simulink model "F16ASYM_Controlled"  (R2015a)
settings: Solver=ode3  SolverMode=SingleTasking  StartTime=0.0  StopTime=inf  FixedStep=T_sim  RelTol=1e-3
InitFcn:
  | load('NN_c_weights_Last_stable.mat')
StopFcn:
  | Final_results
values from neighbouring files (symbols this model uses):
  a1 = fitresult.p1    [Stall_protection.m]
  alpha_map_eval = ones(size(M_eval))*NaN    [Auto_trim_aid.m]    (also in Autotrim_maps.mat = [nan nan 0.277598136245 0.119432432992 0.0579479097061 0.027)
  beta_map_eval = ones(size(M_eval))*NaN    [Auto_trim_aid.m]    (also in Autotrim_maps.mat = [nan nan -0.00151549403324 0.00117807579006 -0.0052086799721)
  C_L_0 = fitresult.p2    [Stall_protection.m]
  G_eval = NaN*ones(size(M_sq,2),size(H_sq,2))    [Stall_protection.m]
  H_sq = unique(sort(H_sq))    [Stall_protection.m]
  H_sq_autotrim = min( F_envelope.H_1g):2000:max(F_envelope.H_1g)    [Auto_trim_aid.m]    (also in Autotrim_maps.mat = [0 2000 4000 6000 8000 10000 12000 14000 16000 18000])
  K_b_q_extrap_ACC = K_b_q_extrap    [RUN_ME.m]
  K_b_q_extrap_AoA = K_b_q_extrap    [RUN_ME.m]
  M_sq = unique(sort(M_sq))    [Stall_protection.m]
  M_sq_autotrim = 0:0.1:max(F_envelope.M_1g)    [Auto_trim_aid.m]    (also in Autotrim_maps.mat = [0 0.1 0.2 0.3 0.4 0.5 0.6 0.7 0.8 0.9 1 1.1 ... (21 element)
  T_sim = 0.02    [RUN_ME.m]
  tau_q_extrap_ACC = tau_q_extrap    [RUN_ME.m]
  tau_q_extrap_AoA = tau_q_extrap    [RUN_ME.m]
  velocity = M_eval(I,J)*a    [Auto_trim_aid.m]
undefined symbols (not defined in the file or in its folder): ACCEL, B, Earth, fi_flag_Simulink, GYRO, H_sq_sche, k_B, K_b_ACC_extrap, K_b_AoA_extrap, latitude, longitude, m, m_B, M_sq_sche, Model_used_flag, rad, s, sigbuilder_block, Stall_curve, tau_ACC_extrap, tau_AoA_extrap, Theta_1_roll_last, Theta_2_roll_last, Theta_3_roll_last, trim_control, trim_state, trim_throttle, V_Comp_A_w_z_last, V_Comp_last, V_Comp_last_ONE, V_long_lastA_w_z, V_long_lastAoA, V_roll_last, V_roll_lastMOD, V_yaw_last, W_Comp_A_w_z_last, W_Comp_last, W_long_lastA_w_z, W_long_lastAoA, W_roll_last, W_roll_lastMOD, W_yaw_last, WGS84
libraries: Adaptive_FaultTolerantControl x57, dspsigops x37, F16_Actuator_Library x14, commnoisgen2 x13, simulink x11, simulink_extras x10, dsparch4 x6, aerolibatmos2 x6, aerolibtransform2 x6, aerolibfltsims x3, dspvision x3, dspsnks4 x3
(part 3 of 14)

== system F16ASYM_Controlled/NDI/NDI: NO RECONFIG ==
  note: These two block MUST be evaluated at the same dynamics X
      | and control deflections delta*
      |
      |
      | delta* are a given set of control deflection: can be either the initial trim set
      | or the previous deflections
  Est reconf : Inport
  Angular_acc_des (rad/s^2) : Inport  Port=2
  All_meas : Inport  Port=3
  Control_defl for eval : Inport  Port=4
  Bus Selector : BusSelector  OutputSignals=signal1.omega_b meas (rad/s),signal2.q (Pa),signal1.Alt meas (m),signal1.V_TAS (m/s),signal1.AoA meas (rad),signal1.SS meas (rad),signal1.Throttle_meas
  Demux : Demux  Outputs=3
  Dim_less : Subsystem
  Inversion : Sum  Inputs=|+-
  Memory : Memory  X0=[0,0,0]
  Mom Coefficients gradient with control deflections at the given dynamics X: It performs perturbations theory arroun the given control deflections : MATLABFcn  MATLABFcn=Moms_Coeff_Grad_estimator  OutputDimensions=21  OutputSignalType=real
  Mux : Mux  Inputs=3
  Mux1 : Mux  Inputs=7
  Pre-Inverter : MATLAB Function  TreatAsAtomicUnit=on
  Reshape : Reshape  OutputDimensionality=Customize  OutputDimensions=[k_B,m_B]
  Terminator : Terminator
  Trim controls Asym In LEFs: Additionaly from dLEF : Constant  Commented=on  Value=[trim_control(1),trim_control(1),trim_control(2),-trim_control(2),trim_control(3),0,0]
  "f(x)  Mom Coefficients due to the dynamics: Coefficients model with control inputs " : MATLABFcn  MATLABFcn=Moms_Coeff_estimator  OutputDimensions=3  OutputSignalType=real
  Virtual Control Commands : Outport
  B online : Outport  Port=2
  Control_defl evald : Outport  Port=3
  Mom coef comm : Outport  Port=4
  wires:
  Est reconf/1 -> Terminator/1
  Reshape/1 -> B online/1
  Mom Coefficients gradient with control deflections at the given dynamics X: It performs perturbations theory arroun the given control deflections/1 -> Reshape/1
  Mux/1 -> Memory/1, Inversion/1
  Bus Selector/7 -> Mux1/6  "<Throttle_meas>"
  Mux1/1 -> Mom Coefficients gradient with control deflections at the given dynamics X: It performs perturbations theory arroun the given control deflections/1, "f(x)  Mom Coefficients due to the dynamics: Coefficients model with control inputs "/1
  Control_defl for eval/1 -> Mux1/7, Control_defl evald/1
  Bus Selector/6 -> Mux1/4  "<SS meas (rad)>"
  Bus Selector/5 -> Mux1/3  "<AoA meas (rad)>"
  Bus Selector/4 -> Mux1/2  "<V_TAS (m/s)>"
  Bus Selector/3 -> Mux1/1  "<Alt meas (m)>"
  "f(x)  Mom Coefficients due to the dynamics: Coefficients model with control inputs "/1 -> Inversion/2  "f(x) or C_x"
  Dim_less/3(C_N des) -> Mux/3
  Dim_less/2(C_M des) -> Mux/2
  Dim_less/1(C_L des) -> Mux/1
  Pre-Inverter/3(N_comm) -> Dim_less/3(N_comm)
  Pre-Inverter/2(M_comm) -> Dim_less/2(M_comm)
  Pre-Inverter/1(L_comm) -> Dim_less/1(L_comm)
  Bus Selector/2 -> Dim_less/4(q)  "<q (Pa)>"
  All_meas/1 -> Bus Selector/1
  Demux/1 -> Pre-Inverter/1(p_dot_comm)
  Demux/3 -> Pre-Inverter/3(r_dot_comm)
  Demux/2 -> Pre-Inverter/2(q_dot_comm)
  Angular_acc_des (rad/s^2)/1 -> Demux/1
  Bus Selector/1 -> Mux1/5, Pre-Inverter/4(omega_b)  "<omega_b meas (rad/s)>"
  Inversion/1 -> Virtual Control Commands/1
  Memory/1 -> Mom coef comm/1

== system F16ASYM_Controlled/NDI/NDI: RECONFIG ==
  note: These two block MUST be evaluated at the same dynamics X
      | and control deflections delta*
      |
      |
      | delta* are a given set of control deflection: can be either the initial trim set
      | or the previous deflections
  note: INPUTS
      | States:
      |
      | 1. Altitude
      | 2. TAS velocity
      | 3. alpha in rad
      | 4. beta in rads
      | 5. P
      | 6. Q
      | 7. R
      | 8. Throttle
      | 9. Elevator_L in deg
      | 10. Elevator_R in deg
      | 11. Aileron_L
      | 12. Aileron_R
      | 13. Rudder
      | 14. LEF_L
      | 15. LEF_R
      |
      | RECONFIGURATION PARAMETERS
      |
      | 16. mass  Estimated mass
      | 17. S_current_L
      | 18. S_current_R
      | 19. S_fin_current
      | 20. x_cg
      | 21. Jy
      | 22. Jxz
      | 23. Jz
      | 24. Jx
      | 25. EFF_el_L
      | 26. EFF_el_R
      | 27. EFF_ail_L
      | 28 EFF_ail_R
      | 29. EFF_rud
      | 30. EFF_lef_L
      | 31. EFF_lef_R
      | 32. Delta_C_Lift_X
      | 33. Delta_C_Drag_X
      | 34. Delta_C_m_X
  Est reconf : Inport
  Angular_acc_des (rad/s^2) : Inport  Port=2
  All_meas : Inport  Port=3
  Control_defl for eval : Inport  Port=4
  Bus Selector : BusSelector  OutputSignals=signal1.omega_b meas (rad/s),signal2.q (Pa),signal1.Alt meas (m),signal1.V_TAS (m/s),signal1.AoA meas (rad),signal1.SS meas (rad),signal1.Throttle_meas
  Bus Selector1 : BusSelector  OutputSignals=Reconfig signal
  Controls : Scope
      settings: SaveName=ScopeData19
  Demux : Demux  Outputs=3
  Dim_less : Subsystem
  Inversion : Sum  Inputs=|+-
  Memory : Memory  X0=[0,0,0]
  Mom Coefficients gradient with control deflections at the given dynamics X: It performs perturbations theory arroun the given control deflections : MATLABFcn  MATLABFcn=Moms_Coeff_Grad_Reconf_estimator  OutputDimensions=21  OutputSignalType=real
  Mux : Mux  Inputs=3
  Mux1 : Mux  Inputs=7
  Mux2 : Mux  Inputs=[15 19]
  Plant : Scope
      settings: SaveName=ScopeData11
  Pre-Inverter : MATLAB Function  TreatAsAtomicUnit=on
  Reshape : Reshape  OutputDimensionality=Customize  OutputDimensions=[k_B,m_B]
  Signal Specification : SignalSpecification  Dimensions=19
  Trim controls Asym In LEFs: Additionaly from dLEF : Constant  Commented=on  Value=[trim_control(1),trim_control(1),trim_control(2),-trim_control(2),trim_control(3),0,0]
  f(x)  Mom Coefficients due to the dynamics: Coefficients model with control inputs : MATLABFcn  MATLABFcn=Moms_Coeff_Reconf_estimator  OutputDimensions=3  OutputSignalType=real
  Virtual Control Commands : Outport
  B online : Outport  Port=2
  Control_defl evald : Outport  Port=3
  Mom coef comm : Outport  Port=4
  wires:
  Inversion/1 -> Controls/1, Virtual Control Commands/1
  Bus Selector/1 -> Pre-Inverter/4(omega_b), Mux1/5  "<omega_b meas (rad/s)>"
  Angular_acc_des (rad/s^2)/1 -> Demux/1
  Demux/2 -> Pre-Inverter/2(q_dot_comm)
  Demux/3 -> Pre-Inverter/3(r_dot_comm)
  Demux/1 -> Pre-Inverter/1(p_dot_comm)
  All_meas/1 -> Bus Selector/1
  Bus Selector/2 -> Dim_less/4(q)  "<q (Pa)>"
  Pre-Inverter/1(L_comm) -> Dim_less/1(L_comm)
  Pre-Inverter/2(M_comm) -> Dim_less/2(M_comm)
  Pre-Inverter/3(N_comm) -> Dim_less/3(N_comm)
  Dim_less/1(C_L des) -> Mux/1
  Dim_less/2(C_M des) -> Mux/2
  Dim_less/3(C_N des) -> Mux/3
  f(x)  Mom Coefficients due to the dynamics: Coefficients model with control inputs/1 -> Plant/1, Inversion/2  "f(x) or C_x"
  Bus Selector/3 -> Mux1/1  "<Alt meas (m)>"
  Bus Selector/4 -> Mux1/2  "<V_TAS (m/s)>"
  Bus Selector/5 -> Mux1/3  "<AoA meas (rad)>"
  Bus Selector/6 -> Mux1/4  "<SS meas (rad)>"
  Control_defl for eval/1 -> Mux1/7, Control_defl evald/1
  Bus Selector/7 -> Mux1/6  "<Throttle_meas>"
  Mux/1 -> Inversion/1, Memory/1
  Mom Coefficients gradient with control deflections at the given dynamics X: It performs perturbations theory arroun the given control deflections/1 -> Reshape/1
  Reshape/1 -> B online/1
  Est reconf/1 -> Bus Selector1/1
  Bus Selector1/1 -> Signal Specification/1  "<Reconfig signal>"
  Mux1/1 -> Mux2/1
  Mux2/1 -> Mom Coefficients gradient with control deflections at the given dynamics X: It performs perturbations theory arroun the given control deflections/1, f(x)  Mom Coefficients due to the dynamics: Coefficients model with control inputs/1
  Signal Specification/1 -> Mux2/2
  Memory/1 -> Mom coef comm/1

== system F16ASYM_Controlled/Primary Controller/P con  + Crossed NN + AWU+Lim + hand-over+Scheduling ==
  note: Indicator correspond to 0
  note: Indicator correspond to 1
  A_w_z des : Inport
  AoA des (rad) : Inport  Port=2
  p des (rad/s) : Inport  Port=3
  beta des (rad) : Inport  Port=4
  Anti-windup A_w_z : Inport  Port=5
  Anti-windup AoA : Inport  Port=6
  Anti-windup beta : Inport  Port=7
  All measures : Inport  Port=8
  Anti-windup signals : Inport  Port=9
  A_w_z des1 : InportShadow
  Anti-windup A_w_z1 : InportShadow  Port=5
  Anti-windup AoA1 : InportShadow  Port=6
  Anti-windup beta1 : InportShadow  Port=7
  Anti-windup signals1 : InportShadow  Port=9
  AoA des (rad)1 : InportShadow  Port=2
  Bus Selector : BusSelector  OutputSignals=signal2.a,signal1.V_TAS (m/s)
  Gain2 : Gain  Gain=2
  Logical Operator : Logic  Operator=NOT  IconShape=distinctive  AllPortsSameDT=off  OutDataTypeStr=boolean
  Min TAS : Product  Inputs=**
  "P controller + adaptive Crossed NN + AWU+Lim    in ACC " : Subsystem  VariantControl=Adaptive Controller Crossed+AWU+Lim
  P controller + adaptive Crossed NN + AWU+Lim   in AoA : Subsystem  VariantControl=Adaptive Controller Crossed+AWU+Lim
  Relational Operator5 : RelationalOperator  OutDataTypeStr=boolean
  "Transitions Smoother " : Subsystem
  beta des (rad)1 : InportShadow  Port=4
  p des (rad/s)1 : InportShadow  Port=3
  Angular acc des : Outport
  Control_in : Outport  Port=2
  wires:
  Logical Operator/1 -> "P controller + adaptive Crossed NN + AWU+Lim    in ACC "/10(Active)
  "Transitions Smoother "/1(Ang accels comm) -> Angular acc des/1
  Relational Operator5/1 -> P controller + adaptive Crossed NN + AWU+Lim   in AoA/10(Active), Control_in/1, "Transitions Smoother "/2(Indicator), Logical Operator/1
  P controller + adaptive Crossed NN + AWU+Lim   in AoA/1(Angular acc des) -> "Transitions Smoother "/1(From AoA)
  "P controller + adaptive Crossed NN + AWU+Lim    in ACC "/1(Angular acc des) -> "Transitions Smoother "/3(From  ACC)
  Bus Selector/2 -> Relational Operator5/2  "<V_TAS (m/s)>"
  Gain2/1 -> Relational Operator5/1
  Min TAS/1 -> Gain2/1
  Bus Selector/1 -> Min TAS/2  "<a>"
  [Min_Mach] -> Min TAS/1  "Min M"
  Anti-windup signals1/1 -> "P controller + adaptive Crossed NN + AWU+Lim    in ACC "/9(Anti-windup signals)
  All measures/1 -> P controller + adaptive Crossed NN + AWU+Lim   in AoA/8(All measures), Bus Selector/1, "P controller + adaptive Crossed NN + AWU+Lim    in ACC "/8(All measures)
  Anti-windup beta1/1 -> "P controller + adaptive Crossed NN + AWU+Lim    in ACC "/7(Anti-windup beta)
  Anti-windup AoA1/1 -> "P controller + adaptive Crossed NN + AWU+Lim    in ACC "/6(Anti-windup AoA)
  Anti-windup A_w_z1/1 -> "P controller + adaptive Crossed NN + AWU+Lim    in ACC "/5(Anti-windup A_w_z)
  beta des (rad)1/1 -> "P controller + adaptive Crossed NN + AWU+Lim    in ACC "/4(beta des (rad))
  p des (rad/s)1/1 -> "P controller + adaptive Crossed NN + AWU+Lim    in ACC "/3(p des (rad/s))
  AoA des (rad)1/1 -> "P controller + adaptive Crossed NN + AWU+Lim    in ACC "/2(AoA des (rad))
  A_w_z des1/1 -> "P controller + adaptive Crossed NN + AWU+Lim    in ACC "/1(A_w_z des)
  p des (rad/s)/1 -> P controller + adaptive Crossed NN + AWU+Lim   in AoA/3(p des (rad/s))
  beta des (rad)/1 -> P controller + adaptive Crossed NN + AWU+Lim   in AoA/4(beta des (rad))
  AoA des (rad)/1 -> P controller + adaptive Crossed NN + AWU+Lim   in AoA/2(AoA des (rad))
  Anti-windup AoA/1 -> P controller + adaptive Crossed NN + AWU+Lim   in AoA/6(Anti-windup AoA)
  Anti-windup A_w_z/1 -> P controller + adaptive Crossed NN + AWU+Lim   in AoA/5(Anti-windup A_w_z)
  A_w_z des/1 -> P controller + adaptive Crossed NN + AWU+Lim   in AoA/1(A_w_z des)
  Anti-windup beta/1 -> P controller + adaptive Crossed NN + AWU+Lim   in AoA/7(Anti-windup beta)
  Anti-windup signals/1 -> P controller + adaptive Crossed NN + AWU+Lim   in AoA/9(Anti-windup signals)

== system F16ASYM_Controlled/Primary Controller/P con + Crossed NN + AWU+Lim + hand-over ==
  note: Indicator correspond to 1
  note: Indicator correspond to 0
  A_w_z des : Inport
  AoA des (rad) : Inport  Port=2
  p des (rad/s) : Inport  Port=3
  beta des (rad) : Inport  Port=4
  Anti-windup A_w_z : Inport  Port=5
  Anti-windup AoA : Inport  Port=6
  Anti-windup beta : Inport  Port=7
  All measures : Inport  Port=8
  Anti-windup signals : Inport  Port=9
  A_w_z des1 : InportShadow
  Anti-windup A_w_z1 : InportShadow  Port=5
  Anti-windup AoA1 : InportShadow  Port=6
  Anti-windup beta1 : InportShadow  Port=7
  Anti-windup signals1 : InportShadow  Port=9
  AoA des (rad)1 : InportShadow  Port=2
  Bus Selector : BusSelector  OutputSignals=signal2.a,signal1.V_TAS (m/s)
  Gain2 : Gain  Gain=2
  Logical Operator : Logic  Operator=NOT  IconShape=distinctive  AllPortsSameDT=off  OutDataTypeStr=boolean
  Min TAS : Product  Inputs=**
  "P controller + adaptive Crossed NN + AWU+Lim    in ACC " : Subsystem  VariantControl=Adaptive Controller Crossed+AWU+Lim
  P controller + adaptive Crossed NN + AWU+Lim   in AoA : Subsystem  VariantControl=Adaptive Controller Crossed+AWU+Lim
  Relational Operator5 : RelationalOperator  OutDataTypeStr=boolean
  Scope : Scope
      settings: YMin=-2.75  YMax=0.25  SaveName=ScopeData32
  Scope1 : Scope  Commented=on
      settings: YMin=-2.75  YMax=0.25  SaveName=ScopeData33
  Switch : Switch  Commented=on  Threshold=0.5  InputSameDT=on
  Transition smoother : MATLAB Function  Commented=on  TreatAsAtomicUnit=on
  "Transitions Smoother " : Subsystem
  Transitions Smotother 1 : Subsystem  Commented=on
  Unit Delay : UnitDelay  Commented=on  SampleTime=-1
  beta des (rad)1 : InportShadow  Port=4
  p des (rad/s)1 : InportShadow  Port=3
  Angular acc des : Outport
  Control_in : Outport  Port=2
  wires:
  Anti-windup signals/1 -> P controller + adaptive Crossed NN + AWU+Lim   in AoA/9(Anti-windup signals)
  Anti-windup beta/1 -> P controller + adaptive Crossed NN + AWU+Lim   in AoA/7(Anti-windup beta)
  A_w_z des/1 -> P controller + adaptive Crossed NN + AWU+Lim   in AoA/1(A_w_z des)
  Anti-windup A_w_z/1 -> P controller + adaptive Crossed NN + AWU+Lim   in AoA/5(Anti-windup A_w_z)
  Anti-windup AoA/1 -> P controller + adaptive Crossed NN + AWU+Lim   in AoA/6(Anti-windup AoA)
  AoA des (rad)/1 -> P controller + adaptive Crossed NN + AWU+Lim   in AoA/2(AoA des (rad))
  beta des (rad)/1 -> P controller + adaptive Crossed NN + AWU+Lim   in AoA/4(beta des (rad))
  p des (rad/s)/1 -> P controller + adaptive Crossed NN + AWU+Lim   in AoA/3(p des (rad/s))
  A_w_z des1/1 -> "P controller + adaptive Crossed NN + AWU+Lim    in ACC "/1(A_w_z des)
  AoA des (rad)1/1 -> "P controller + adaptive Crossed NN + AWU+Lim    in ACC "/2(AoA des (rad))
  p des (rad/s)1/1 -> "P controller + adaptive Crossed NN + AWU+Lim    in ACC "/3(p des (rad/s))
  beta des (rad)1/1 -> "P controller + adaptive Crossed NN + AWU+Lim    in ACC "/4(beta des (rad))
  Anti-windup A_w_z1/1 -> "P controller + adaptive Crossed NN + AWU+Lim    in ACC "/5(Anti-windup A_w_z)
  Anti-windup AoA1/1 -> "P controller + adaptive Crossed NN + AWU+Lim    in ACC "/6(Anti-windup AoA)
  Anti-windup beta1/1 -> "P controller + adaptive Crossed NN + AWU+Lim    in ACC "/7(Anti-windup beta)
  All measures/1 -> "P controller + adaptive Crossed NN + AWU+Lim    in ACC "/8(All measures), Bus Selector/1, P controller + adaptive Crossed NN + AWU+Lim   in AoA/8(All measures)
  Anti-windup signals1/1 -> "P controller + adaptive Crossed NN + AWU+Lim    in ACC "/9(Anti-windup signals)
  [Min_Mach] -> Min TAS/1  "Min M"
  Bus Selector/1 -> Min TAS/2  "<a>"
  Min TAS/1 -> Gain2/1
  Gain2/1 -> Relational Operator5/1
  Bus Selector/2 -> Relational Operator5/2  "<V_TAS (m/s)>"
  "P controller + adaptive Crossed NN + AWU+Lim    in ACC "/1(Angular acc des) -> "Transitions Smoother "/3(From  ACC)
  P controller + adaptive Crossed NN + AWU+Lim   in AoA/1(Angular acc des) -> "Transitions Smoother "/1(From AoA)
  Relational Operator5/1 -> Logical Operator/1, Control_in/1, "Transitions Smoother "/2(Indicator), P controller + adaptive Crossed NN + AWU+Lim   in AoA/10(Active)
  Transition smoother/2(indicator_out) -> Unit Delay/1
  Unit Delay/1 -> Transition smoother/4(indicator_prev)
  "Transitions Smoother "/1(Ang accels comm) -> Angular acc des/1, Scope/1
  Switch/1 -> Scope1/1
  Logical Operator/1 -> "P controller + adaptive Crossed NN + AWU+Lim    in ACC "/10(Active)

== system F16ASYM_Controlled/Primary Controller/P con + adaptive Crossed NN + AWU+Lim + Scheduling ==
  A_w_z des : Inport
  AoA des (rad) : Inport  Port=2
  p des (rad/s) : Inport  Port=3
  beta des (rad) : Inport  Port=4
  Anti-windup A_w_z : Inport  Port=5
  Anti-windup AoA : Inport  Port=6
  Anti-windup beta : Inport  Port=7
  All measures : Inport  Port=8
  Anti-windup signals : Inport  Port=9
  Body Rates Controller : Subsystem  Variant=on  OverrideUsingVariant=Body rates controller of AoA
  Bus Creator : BusCreator  Inputs=3
  Bus Creator1 : BusCreator  Inputs=3
  Bus Creator2 : BusCreator
  Bus Creator3 : BusCreator  Inputs=2
  Bus Selector3 : BusSelector  OutputSignals=signal1.SS meas (rad)
  Complete crossed On-line (adaptive) multi-layer NN : Subsystem  Variant=on  OverrideUsingVariant=NN on AoA
      mask Display:
      | image(imread('ANN.png'))
      | 
      | port_label('input', 1, 'v prev')
      | port_label('input', 2, 'All meas')
      | port_label('input', 3, 'NN vars')
      | port_label('input', 4, 'Anti-windup')
      | 
      | port_label('output', 1, 'v_ad^')
  Constant : Constant  Value=NaN
  Display{,1..3,5..6} (6 alike) : Display
  "Display4 " : Display
  Lat_dir Dyn Inversion: beta_dot->r_c : Subsystem
  Long Dyn Inversion: alpha_dot ->q : Subsystem
  Longitudinal Controller: AoA or A_w_z : Subsystem  Variant=on  OverrideUsingVariant=Controller of AoA
  Memory : Memory  X0=[0,0,0]
  Physical limitation : Subsystem
  Ref Model and P Controller : Adaptive_FaultTolerantControl/Ref Model and P Controller  tau=0.45  y_i=trim_state(9)  K_f=1  K_b=5
  Scope1 : Scope
      settings: TimeRange=18  YMax=25  SaveName=ScopeData27
  Scope2 : Scope
      settings: TimeRange=18  YMax=25  SaveName=ScopeData7
  Scope3 : Scope
      settings: TimeRange=18  YMin=-20  YMax=1  SaveName=ScopeData21
  "Sigmoid " : Subsystem  mask{a=0.15}
      mask prompts: a "Sigmoid a param"
      mask TypeOptions a: a/Value
      mask Display:
      | x=-25:0.1:25;
      | 
      | y=(2.0 ./ (1.0 + exp(-a.*x))-1) ;
      | y2=zeros(size(x));
      | 
      | plot(x,y,x,y2);
      | 
      | text(-12,0.5, ['a= ',num2str(a)])
  Sum : Sum  Inputs=-+|
  Sum1 : Sum  Inputs=+-|
  Terminator1 : Terminator
  To Workspace : ToWorkspace  VariableName=Comm_ang_accel  SaveFormat=Timeseries  SampleTime=-1
  To Workspace1 : ToWorkspace  VariableName=NN_action  SaveFormat=Timeseries  SampleTime=-1
  Angular acc des : Outport
  Control_in : Outport  Port=2
  wires:
  Constant/1 -> Control_in/1
  Physical limitation/1(v limted) -> Angular acc des/1
  Anti-windup signals/1 -> Complete crossed On-line (adaptive) multi-layer NN/4(AWU)
  Ref Model and P Controller/1 -> Lat_dir Dyn Inversion: beta_dot->r_c/1(beta_dot_c), Display5/1
  Complete crossed On-line (adaptive) multi-layer NN/1(v_ad^) -> To Workspace1/1, Sum/1, Display2/1, Scope1/1  "v_ad^"
  "Sigmoid "/1(Out) -> Memory/1
  Anti-windup beta/1 -> Terminator1/1
  Bus Creator3/1 -> Bus Creator/3  "beta_r_chanel"
  Bus Creator2/1 -> Bus Creator3/2  "beta_chanel vars"
  Body Rates Controller/3(r_chanel vars) -> Bus Creator3/1  "r_chanel vars"
  Ref Model and P Controller/5 -> Bus Creator2/4  "K_b_beta"
  Ref Model and P Controller/4 -> Sum1/2
  Sum1/1 -> Bus Creator2/3  "beta_err"
  Ref Model and P Controller/3 -> Bus Creator2/2, Sum1/1  "beta_sf"
  Ref Model and P Controller/2 -> Bus Creator2/1  "beta_sf_dot"
  Bus Creator1/1 -> Bus Creator/1  "Long chanel"
  Longitudinal Controller: AoA or A_w_z/2(alpha_chanel vars) -> Bus Creator1/2  "alpha_chanel vars"
  Longitudinal Controller: AoA or A_w_z/1(A_chanel vars) -> Bus Creator1/1  "A_chanel vars"
  Body Rates Controller/1(q_chanel vars) -> Bus Creator1/3  "q_chanel_vars"
  Body Rates Controller/2(p_chanel vars) -> Bus Creator/2  "p_chanel_vars"
  Memory/1 -> Complete crossed On-line (adaptive) multi-layer NN/1(v_ad^ prev)
  Bus Creator/1 -> Complete crossed On-line (adaptive) multi-layer NN/3(NN variables)
  Body Rates Controller/4(Angular acc des (rad/s^2)) -> Scope2/1, Sum/2, Display3/1  "v_p+v_dot_ff"
  All measures/1 -> Longitudinal Controller: AoA or A_w_z/5(All meas), Long Dyn Inversion: alpha_dot ->q/2(All_meas), Bus Selector3/1, Lat_dir Dyn Inversion: beta_dot->r_c/2(All_meas), Body Rates Controller/4(All_meas), Physical limitation/2(all meas), Complete crossed On-line (adaptive) multi-layer NN/2(All_meas)
  Sum/1 -> To Workspace/1, Scope3/1, Physical limitation/1(v comm), "Sigmoid "/1(In), "Display4 "/1  "v"
  A_w_z des/1 -> Longitudinal Controller: AoA or A_w_z/1(A_w_z des)
  Anti-windup A_w_z/1 -> Longitudinal Controller: AoA or A_w_z/3(Anti-windup A_w_z)
  Anti-windup AoA/1 -> Longitudinal Controller: AoA or A_w_z/4(Anti-windup AoA)
  AoA des (rad)/1 -> Longitudinal Controller: AoA or A_w_z/2(AoA des (rad))
  Longitudinal Controller: AoA or A_w_z/3(alpha_dot_c) -> Display/1, Long Dyn Inversion: alpha_dot ->q/1(alpha_dot_c)
  beta des (rad)/1 -> Ref Model and P Controller/1
  Long Dyn Inversion: alpha_dot ->q/1(q_c) -> Display1/1, Body Rates Controller/2(q_ref)
  p des (rad/s)/1 -> Body Rates Controller/1(p_ref)
  Bus Selector3/1 -> Ref Model and P Controller/2  "<SS meas (rad)>"
  Lat_dir Dyn Inversion: beta_dot->r_c/1(r_c) -> Body Rates Controller/3(r_ref), Display6/1

== system F16ASYM_Controlled/Primary Controller/P cont + adaptive Crossed NN + AWU+Lim  ==
  A_w_z des : Inport
  AoA des (rad) : Inport  Port=2
  p des (rad/s) : Inport  Port=3
  beta des (rad) : Inport  Port=4
  Anti-windup A_w_z : Inport  Port=5
  Anti-windup AoA : Inport  Port=6
  Anti-windup beta : Inport  Port=7
  All measures : Inport  Port=8
  Anti-windup signals : Inport  Port=9
  Body Rates Controller : Subsystem
  Bus Creator : BusCreator  Inputs=3
  Bus Creator1 : BusCreator  Inputs=3
  Bus Creator2 : BusCreator
  Bus Creator3 : BusCreator  Inputs=2
  Bus Selector3 : BusSelector  OutputSignals=signal1.SS meas (rad)
  Complete crossed On-line (adaptive) multi-layer NN : Subsystem  Variant=on  OverrideUsingVariant=NN on AoA
      mask Display:
      | image(imread('ANN.png'))
      | 
      | port_label('input', 1, 'v prev')
      | port_label('input', 2, 'All meas')
      | port_label('input', 3, 'NN vars')
      | port_label('input', 4, 'Anti-windup')
      | 
      | port_label('output', 1, 'v_ad^')
  Constant : Constant  Value=NaN
  Display{,1..3,5..6} (6 alike) : Display
  "Display4 " : Display
  Lat_dir Dyn Inversion: beta_dot->r_c : Subsystem
  Long Dyn Inversion: alpha_dot ->q : Subsystem
  Longitudinal Controller: AoA or A_w_z : Subsystem  Variant=on  OverrideUsingVariant=Controller of AoA
  Memory : Memory  X0=[0,0,0]
  Physical limitation : Subsystem
  Ref Model and P Controller : Adaptive_FaultTolerantControl/Ref Model and P Controller  tau=0.8  y_i=trim_state(9)  K_f=1  K_b=5
  Scope1 : Scope
      settings: TimeRange=35  YMin=-0.0025  YMax=0.0275  SaveName=ScopeData27
  "Sigmoid " : Subsystem  mask{a=0.15}
      mask prompts: a "Sigmoid a param"
      mask TypeOptions a: a/Value
      mask Display:
      | x=-25:0.1:25;
      | 
      | y=(2.0 ./ (1.0 + exp(-a.*x))-1) ;
      | y2=zeros(size(x));
      | 
      | plot(x,y,x,y2);
      | 
      | text(-12,0.5, ['a= ',num2str(a)])
  Sum : Sum  Inputs=-+|
  Sum1 : Sum  Inputs=+-|
  Terminator1 : Terminator
  To Workspace : ToWorkspace  VariableName=NN_output  SaveFormat=Timeseries  SampleTime=-1
  To Workspace1 : ToWorkspace  VariableName=Comm_ang_acce  SaveFormat=Timeseries  SampleTime=-1
  Angular acc des : Outport
  Control_in : Outport  Port=2
  wires:
  Lat_dir Dyn Inversion: beta_dot->r_c/1(r_c) -> Display6/1, Body Rates Controller/3(r_ref)
  Bus Selector3/1 -> Ref Model and P Controller/2  "<SS meas (rad)>"
  p des (rad/s)/1 -> Body Rates Controller/1(p_ref)
  Long Dyn Inversion: alpha_dot ->q/1(q_c) -> Body Rates Controller/2(q_ref), Display1/1
  beta des (rad)/1 -> Ref Model and P Controller/1
  Longitudinal Controller: AoA or A_w_z/3(alpha_dot_c) -> Long Dyn Inversion: alpha_dot ->q/1(alpha_dot_c), Display/1
  AoA des (rad)/1 -> Longitudinal Controller: AoA or A_w_z/2(AoA des (rad))
  Anti-windup AoA/1 -> Longitudinal Controller: AoA or A_w_z/4(Anti-windup AoA)
  Anti-windup A_w_z/1 -> Longitudinal Controller: AoA or A_w_z/3(Anti-windup A_w_z)
  A_w_z des/1 -> Longitudinal Controller: AoA or A_w_z/1(A_w_z des)
  Sum/1 -> To Workspace1/1, "Display4 "/1, "Sigmoid "/1(In), Physical limitation/1(v comm)  "v"
  All measures/1 -> Complete crossed On-line (adaptive) multi-layer NN/2(All_meas), Physical limitation/2(all meas), Body Rates Controller/4(All_meas), Lat_dir Dyn Inversion: beta_dot->r_c/2(All_meas), Bus Selector3/1, Long Dyn Inversion: alpha_dot ->q/2(All_meas), Longitudinal Controller: AoA or A_w_z/5(All meas)
  Body Rates Controller/4(Angular acc des (rad/s^2)) -> Display3/1, Sum/2  "v_p+v_dot_ff"
  Bus Creator/1 -> Complete crossed On-line (adaptive) multi-layer NN/3(NN variables)
  Memory/1 -> Complete crossed On-line (adaptive) multi-layer NN/1(v_ad^ prev)
  Body Rates Controller/2(p_chanel vars) -> Bus Creator/2  "p_chanel_vars"
  Body Rates Controller/1(q_chanel vars) -> Bus Creator1/3  "q_chanel_vars"
  Longitudinal Controller: AoA or A_w_z/1(A_chanel vars) -> Bus Creator1/1  "A_chanel vars"
  Longitudinal Controller: AoA or A_w_z/2(alpha_chanel vars) -> Bus Creator1/2  "alpha_chanel vars"
  Bus Creator1/1 -> Bus Creator/1  "Long chanel"
  Ref Model and P Controller/2 -> Bus Creator2/1  "beta_sf_dot"
  Ref Model and P Controller/3 -> Sum1/1, Bus Creator2/2  "beta_sf"
  Sum1/1 -> Bus Creator2/3  "beta_err"
  Ref Model and P Controller/4 -> Sum1/2
  Ref Model and P Controller/5 -> Bus Creator2/4  "K_b_beta"
  Body Rates Controller/3(r_chanel vars) -> Bus Creator3/1  "r_chanel vars"
  Bus Creator2/1 -> Bus Creator3/2  "beta_chanel vars"
  Bus Creator3/1 -> Bus Creator/3  "beta_r_chanel"
  Anti-windup beta/1 -> Terminator1/1
  "Sigmoid "/1(Out) -> Memory/1
  Complete crossed On-line (adaptive) multi-layer NN/1(v_ad^) -> Scope1/1, Display2/1, Sum/1, To Workspace/1  "v_ad^"
  Ref Model and P Controller/1 -> Display5/1, Lat_dir Dyn Inversion: beta_dot->r_c/1(beta_dot_c)
  Anti-windup signals/1 -> Complete crossed On-line (adaptive) multi-layer NN/4(AWU)
  Physical limitation/1(v limted) -> Angular acc des/1
  Constant/1 -> Control_in/1

== system F16ASYM_Controlled/Primary Controller/P cont + adaptive Crossed NN + AWU+Lim ONELAYER ==
  A_w_z des : Inport
  AoA des (rad) : Inport  Port=2
  p des (rad/s) : Inport  Port=3
  beta des (rad) : Inport  Port=4
  Anti-windup A_w_z : Inport  Port=5
  Anti-windup AoA : Inport  Port=6
  Anti-windup beta : Inport  Port=7
  All measures : Inport  Port=8
  Anti-windup signals : Inport  Port=9
  Body Rates Controller : Subsystem
  Bus Creator : BusCreator  Inputs=3
  Bus Creator1 : BusCreator  Inputs=3
  Bus Creator2 : BusCreator
  Bus Creator3 : BusCreator  Inputs=2
  Bus Selector3 : BusSelector  OutputSignals=signal1.SS meas (rad)
  Complete crossed On-line (adaptive) multi-layer NN : Subsystem  Variant=on  OverrideUsingVariant=NN on AoA
      mask Display:
      | image(imread('ANN.png'))
      | 
      | port_label('input', 1, 'v prev')
      | port_label('input', 2, 'All meas')
      | port_label('input', 3, 'NN vars')
      | port_label('input', 4, 'Anti-windup')
      | 
      | port_label('output', 1, 'v_ad^')
  Constant : Constant  Value=NaN
  Display{,1..3,5..6} (6 alike) : Display
  "Display4 " : Display
  Lat_dir Dyn Inversion: beta_dot->r_c : Subsystem
  Long Dyn Inversion: alpha_dot ->q : Subsystem
  Longitudinal Controller: AoA or A_w_z : Subsystem  Variant=on  OverrideUsingVariant=Controller of AoA
  Memory : Memory  X0=[0,0,0]
  Physical limitation : Subsystem
  Ref Model and P Controller : Adaptive_FaultTolerantControl/Ref Model and P Controller  tau=0.8  y_i=trim_state(9)  K_f=1  K_b=5
  Scope1 : Scope
      settings: TimeRange=35  YMin=-0.0025  YMax=0.0275  SaveName=ScopeData27
  "Sigmoid " : Subsystem  mask{a=0.15}
      mask prompts: a "Sigmoid a param"
      mask TypeOptions a: a/Value
      mask Display:
      | x=-25:0.1:25;
      | 
      | y=(2.0 ./ (1.0 + exp(-a.*x))-1) ;
      | y2=zeros(size(x));
      | 
      | plot(x,y,x,y2);
      | 
      | text(-12,0.5, ['a= ',num2str(a)])
  Sum : Sum  Inputs=-+|
  Sum1 : Sum  Inputs=+-|
  Terminator1 : Terminator
  To Workspace : ToWorkspace  VariableName=NN_output  SaveFormat=Timeseries  SampleTime=-1
  To Workspace1 : ToWorkspace  VariableName=Comm_ang_acce  SaveFormat=Timeseries  SampleTime=-1
  Angular acc des : Outport
  Control_in : Outport  Port=2
  wires:
  Lat_dir Dyn Inversion: beta_dot->r_c/1(r_c) -> Display6/1, Body Rates Controller/3(r_ref)
  Bus Selector3/1 -> Ref Model and P Controller/2  "<SS meas (rad)>"
  p des (rad/s)/1 -> Body Rates Controller/1(p_ref)
  Long Dyn Inversion: alpha_dot ->q/1(q_c) -> Body Rates Controller/2(q_ref), Display1/1
  beta des (rad)/1 -> Ref Model and P Controller/1
  Longitudinal Controller: AoA or A_w_z/3(alpha_dot_c) -> Long Dyn Inversion: alpha_dot ->q/1(alpha_dot_c), Display/1
  AoA des (rad)/1 -> Longitudinal Controller: AoA or A_w_z/2(AoA des (rad))
  Anti-windup AoA/1 -> Longitudinal Controller: AoA or A_w_z/4(Anti-windup AoA)
  Anti-windup A_w_z/1 -> Longitudinal Controller: AoA or A_w_z/3(Anti-windup A_w_z)
  A_w_z des/1 -> Longitudinal Controller: AoA or A_w_z/1(A_w_z des)
  Sum/1 -> To Workspace1/1, "Display4 "/1, "Sigmoid "/1(In), Physical limitation/1(v comm)  "v"
  All measures/1 -> Complete crossed On-line (adaptive) multi-layer NN/2(All_meas), Physical limitation/2(all meas), Body Rates Controller/4(All_meas), Lat_dir Dyn Inversion: beta_dot->r_c/2(All_meas), Bus Selector3/1, Long Dyn Inversion: alpha_dot ->q/2(All_meas), Longitudinal Controller: AoA or A_w_z/5(All meas)
  Body Rates Controller/4(Angular acc des (rad/s^2)) -> Display3/1, Sum/2  "v_p+v_dot_ff"
  Bus Creator/1 -> Complete crossed On-line (adaptive) multi-layer NN/3(NN variables)
  Memory/1 -> Complete crossed On-line (adaptive) multi-layer NN/1(v_ad^ prev)
  Body Rates Controller/2(p_chanel vars) -> Bus Creator/2  "p_chanel_vars"
  Body Rates Controller/1(q_chanel vars) -> Bus Creator1/3  "q_chanel_vars"
  Longitudinal Controller: AoA or A_w_z/1(A_chanel vars) -> Bus Creator1/1  "A_chanel vars"
  Longitudinal Controller: AoA or A_w_z/2(alpha_chanel vars) -> Bus Creator1/2  "alpha_chanel vars"
  Bus Creator1/1 -> Bus Creator/1  "Long chanel"
  Ref Model and P Controller/2 -> Bus Creator2/1  "beta_sf_dot"
  Ref Model and P Controller/3 -> Sum1/1, Bus Creator2/2  "beta_sf"
  Sum1/1 -> Bus Creator2/3  "beta_err"
  Ref Model and P Controller/4 -> Sum1/2
  Ref Model and P Controller/5 -> Bus Creator2/4  "K_b_beta"
  Body Rates Controller/3(r_chanel vars) -> Bus Creator3/1  "r_chanel vars"
  Bus Creator2/1 -> Bus Creator3/2  "beta_chanel vars"
  Bus Creator3/1 -> Bus Creator/3  "beta_r_chanel"
  Anti-windup beta/1 -> Terminator1/1
  "Sigmoid "/1(Out) -> Memory/1
  Complete crossed On-line (adaptive) multi-layer NN/1(v_ad^) -> Scope1/1, Display2/1, Sum/1, To Workspace/1  "v_ad^"
  Ref Model and P Controller/1 -> Display5/1, Lat_dir Dyn Inversion: beta_dot->r_c/1(beta_dot_c)
  Anti-windup signals/1 -> Complete crossed On-line (adaptive) multi-layer NN/4(AWU)
  Physical limitation/1(v limted) -> Angular acc des/1
  Constant/1 -> Control_in/1

== system F16ASYM_Controlled/Primary Controller/P controller ==
  A_w_z des : Inport
  AoA des (rad) : Inport  Port=2
  p des (rad/s) : Inport  Port=3
  beta des (rad) : Inport  Port=4
  Anti-windup A_w_z : Inport  Port=5
  Anti-windup AoA : Inport  Port=6
  Anti-windup beta : Inport  Port=7
  All measures : Inport  Port=8
  Anti-windup signals : Inport  Port=9
  Body Rates Controller : Subsystem
  Bus Creator2 : BusCreator
  Bus Selector3 : BusSelector  OutputSignals=signal1.SS meas (rad)
  Constant : Constant  Value=NaN
  Display : Display
  Display1 : Display
  Lat_dir Dyn Inversion: beta_dot->r_c : Subsystem
  Long Dyn Inversion: alpha_dot ->q : Subsystem
  Longitudinal Controller: AoA or A_w_z : Subsystem  Variant=on  OverrideUsingVariant=Controller of AoA
  Ref Model and P Controller : Adaptive_FaultTolerantControl/Ref Model and P Controller  tau=0.8  y_i=trim_state(9)  K_f=1  K_b=5
  Sum1 : Sum  Inputs=+-|
  Terminator : Terminator
  Terminator1 : Terminator
  Terminator2 : Terminator
  Angular acc des : Outport
  Control_in : Outport  Port=2
  wires:
  Anti-windup beta/1 -> Terminator1/1
  Ref Model and P Controller/5 -> Bus Creator2/4  "K_b_beta"
  Ref Model and P Controller/4 -> Sum1/2
  Sum1/1 -> Bus Creator2/3  "beta_err"
  Ref Model and P Controller/3 -> Bus Creator2/2, Sum1/1  "beta_sf"
  Ref Model and P Controller/2 -> Bus Creator2/1  "beta_sf_dot"
  Anti-windup signals/1 -> Terminator/1
  All measures/1 -> Longitudinal Controller: AoA or A_w_z/5(All meas), Long Dyn Inversion: alpha_dot ->q/2(All_meas), Bus Selector3/1, Lat_dir Dyn Inversion: beta_dot->r_c/2(All_meas), Body Rates Controller/4(All_meas)
  A_w_z des/1 -> Longitudinal Controller: AoA or A_w_z/1(A_w_z des)
  Anti-windup A_w_z/1 -> Longitudinal Controller: AoA or A_w_z/3(Anti-windup A_w_z)
  Anti-windup AoA/1 -> Longitudinal Controller: AoA or A_w_z/4(Anti-windup AoA)
  AoA des (rad)/1 -> Longitudinal Controller: AoA or A_w_z/2(AoA des (rad))
  Longitudinal Controller: AoA or A_w_z/3(alpha_dot_c) -> Display/1, Long Dyn Inversion: alpha_dot ->q/1(alpha_dot_c)
  beta des (rad)/1 -> Ref Model and P Controller/1
  Long Dyn Inversion: alpha_dot ->q/1(q_c) -> Body Rates Controller/2(q_ref), Display1/1
  p des (rad/s)/1 -> Body Rates Controller/1(p_ref)
  Ref Model and P Controller/1 -> Lat_dir Dyn Inversion: beta_dot->r_c/1(beta_dot_c)
  Bus Selector3/1 -> Ref Model and P Controller/2  "<SS meas (rad)>"
  Lat_dir Dyn Inversion: beta_dot->r_c/1(r_c) -> Body Rates Controller/3(r_ref)
  Bus Creator2/1 -> Terminator2/1  "beta_chanel vars"
  Body Rates Controller/1(Angular acc des (rad/s^2)) -> Angular acc des/1  "v_p+v_dot_ff"
  Constant/1 -> Control_in/1

== system F16ASYM_Controlled/Primary Controller/P controller + adaptive Crossed NN ==
  A_w_z des : Inport
  AoA des (rad) : Inport  Port=2
  p des (rad/s) : Inport  Port=3
  beta des (rad) : Inport  Port=4
  Anti-windup A_w_z : Inport  Port=5
  Anti-windup AoA : Inport  Port=6
  Anti-windup beta : Inport  Port=7
  All measures : Inport  Port=8
  Anti-windup signals : Inport  Port=9
  Body Rates Controller : Subsystem
  Bus Creator : BusCreator  Inputs=3
  Bus Creator1 : BusCreator  Inputs=3
  Bus Creator2 : BusCreator
  Bus Creator3 : BusCreator  Inputs=2
  Bus Selector3 : BusSelector  OutputSignals=signal1.SS meas (rad)
  Complete crossed On-line (adaptive) multi-layer NN : Subsystem  Variant=on  OverrideUsingVariant=NN on A_w_z
      mask Display:
      | image(imread('ANN.png'))
      | 
      | port_label('input', 1, 'v prev')
      | port_label('input', 2, 'All meas')
      | port_label('input', 3, 'NN vars')
      | 
      | port_label('output', 1, 'v_ad^')
  Display{,1..6} (7 alike) : Display
  Ground : Ground
  Lat_dir Dyn Inversion: beta_dot->r_c : Subsystem
  Long Dyn Inversion: alpha_dot ->q : Subsystem
  Longitudinal Controller: AoA or A_w_z : Subsystem  Variant=on  OverrideUsingVariant=Controller of A_w_z
  Memory : Memory  X0=[0,0,0]
  Ref Model and P Controller : Adaptive_FaultTolerantControl/Ref Model and P Controller  tau=0.45  y_i=trim_state(9)  K_f=1  K_b=5
  "Sigmoid " : Subsystem  mask{a=0.15}
      mask prompts: a "Sigmoid a param"
      mask TypeOptions a: a/Value
      mask Display:
      | x=-25:0.1:25;
      | 
      | y=(2.0 ./ (1.0 + exp(-a.*x))-1) ;
      | y2=zeros(size(x));
      | 
      | plot(x,y,x,y2);
      | 
      | text(-12,0.5, ['a= ',num2str(a)])
  Sum : Sum  Inputs=-+|
  Sum1 : Sum  Inputs=+-|
  Terminator : Terminator
  Terminator1 : Terminator
  Angular acc des : Outport
  Control_in : Outport  Port=2
  wires:
  Anti-windup signals/1 -> Terminator/1
  Ref Model and P Controller/1 -> Lat_dir Dyn Inversion: beta_dot->r_c/1(beta_dot_c), Display5/1
  Complete crossed On-line (adaptive) multi-layer NN/1(v_ad^) -> Display2/1, Sum/1  "v_ad^"
  "Sigmoid "/1(Out) -> Memory/1
  Anti-windup beta/1 -> Terminator1/1
  Bus Creator3/1 -> Bus Creator/3  "beta_r_chanel"
  Bus Creator2/1 -> Bus Creator3/2  "beta_chanel vars"
  Body Rates Controller/3(r_chanel vars) -> Bus Creator3/1  "r_chanel vars"
  Ref Model and P Controller/5 -> Bus Creator2/4  "K_b_beta"
  Ref Model and P Controller/4 -> Sum1/2
  Sum1/1 -> Bus Creator2/3  "beta_err"
  Ref Model and P Controller/3 -> Bus Creator2/2, Sum1/1  "beta_sf"
  Ref Model and P Controller/2 -> Bus Creator2/1  "beta_sf_dot"
  Bus Creator1/1 -> Bus Creator/1  "Long chanel"
  Longitudinal Controller: AoA or A_w_z/2(alpha_chanel vars) -> Bus Creator1/2  "alpha_chanel vars"
  Longitudinal Controller: AoA or A_w_z/1(A_chanel vars) -> Bus Creator1/1  "A_chanel vars"
  Body Rates Controller/1(q_chanel vars) -> Bus Creator1/3  "q_chanel_vars"
  Body Rates Controller/2(p_chanel vars) -> Bus Creator/2  "p_chanel_vars"
  Memory/1 -> Complete crossed On-line (adaptive) multi-layer NN/1(v_ad^ prev)
  Bus Creator/1 -> Complete crossed On-line (adaptive) multi-layer NN/3(NN variables)
  Body Rates Controller/4(Angular acc des (rad/s^2)) -> Sum/2, Display3/1  "v_p+v_dot_ff"
  All measures/1 -> Longitudinal Controller: AoA or A_w_z/5(All meas), Long Dyn Inversion: alpha_dot ->q/2(All_meas), Bus Selector3/1, Lat_dir Dyn Inversion: beta_dot->r_c/2(All_meas), Body Rates Controller/4(All_meas), Complete crossed On-line (adaptive) multi-layer NN/2(All_meas)
  Sum/1 -> Angular acc des/1, "Sigmoid "/1(In), Display4/1  "v"
  A_w_z des/1 -> Longitudinal Controller: AoA or A_w_z/1(A_w_z des)
  Anti-windup A_w_z/1 -> Longitudinal Controller: AoA or A_w_z/3(Anti-windup A_w_z)
  Anti-windup AoA/1 -> Longitudinal Controller: AoA or A_w_z/4(Anti-windup AoA)
  AoA des (rad)/1 -> Longitudinal Controller: AoA or A_w_z/2(AoA des (rad))
  Longitudinal Controller: AoA or A_w_z/3(alpha_dot_c) -> Display/1, Long Dyn Inversion: alpha_dot ->q/1(alpha_dot_c)
  beta des (rad)/1 -> Ref Model and P Controller/1
  Long Dyn Inversion: alpha_dot ->q/1(q_c) -> Body Rates Controller/2(q_ref), Display1/1
  p des (rad/s)/1 -> Body Rates Controller/1(p_ref)
  Bus Selector3/1 -> Ref Model and P Controller/2  "<SS meas (rad)>"
  Lat_dir Dyn Inversion: beta_dot->r_c/1(r_c) -> Body Rates Controller/3(r_ref), Display6/1
  Ground/1 -> Control_in/1

== system F16ASYM_Controlled/Primary Controller/P controller + adaptive Isolated NN ==
  A_w_z des : Inport
  AoA des (rad) : Inport  Port=2
  p des (rad/s) : Inport  Port=3
  beta des (rad) : Inport  Port=4
  Anti-windup A_w_z : Inport  Port=5
  Anti-windup AoA : Inport  Port=6
  Anti-windup beta : Inport  Port=7
  All measures : Inport  Port=8
  Anti-windup signals : Inport  Port=9
  Body Rates Controller : Subsystem
  Bus Creator : BusCreator  Inputs=3
  Bus Creator1 : BusCreator  Inputs=3
  Bus Creator2 : BusCreator
  Bus Creator3 : BusCreator  Inputs=2
  Bus Selector3 : BusSelector  OutputSignals=signal1.SS meas (rad)
  Display{,1..6} (7 alike) : Display
  Ground : Ground
  Lat_dir Dyn Inversion: beta_dot->r_c : Subsystem
  Long Dyn Inversion: alpha_dot ->q : Subsystem
  Longitudinal Controller: AoA or A_w_z : Subsystem  Variant=on  OverrideUsingVariant=Controller of A_w_z
  Memory : Memory  X0=[0,0,0]
  On-line (adaptive) multi-layer NNs : Subsystem
      mask Display:
      | image(imread('ANN.png'))
      | 
      | port_label('input', 1, 'v prev')
      | port_label('input', 2, 'All meas')
      | port_label('input', 3, 'NN vars')
      | 
      | port_label('output', 1, 'v_ad^')
  On-line (adaptive) multi-layer NNs SIMPL : Subsystem  Commented=on
      mask Display:
      | image(imread('ANN.png'))
      | 
      | port_label('input', 1, 'v prev')
      | port_label('input', 2, 'All meas')
      | port_label('input', 3, 'NN vars')
      | 
      | port_label('output', 1, 'v_ad^')
  Ref Model and P Controller : Adaptive_FaultTolerantControl/Ref Model and P Controller  tau=0.45  y_i=trim_state(9)  K_f=1  K_b=5
  "Sigmoid " : Subsystem  mask{a=0.15}
      mask prompts: a "Sigmoid a param"
      mask TypeOptions a: a/Value
      mask Display:
      | x=-25:0.1:25;
      | 
      | y=(2.0 ./ (1.0 + exp(-a.*x))-1) ;
      | y2=zeros(size(x));
      | 
      | plot(x,y,x,y2);
      | 
      | text(-12,0.5, ['a= ',num2str(a)])
  Sum : Sum  Inputs=-+|
  Sum1 : Sum  Inputs=+-|
  Terminator : Terminator
  Terminator1 : Terminator
  Angular acc des : Outport
  Control_in : Outport  Port=2
  wires:
  Lat_dir Dyn Inversion: beta_dot->r_c/1(r_c) -> Display6/1, Body Rates Controller/3(r_ref)
  Bus Selector3/1 -> Ref Model and P Controller/2  "<SS meas (rad)>"
  p des (rad/s)/1 -> Body Rates Controller/1(p_ref)
  Long Dyn Inversion: alpha_dot ->q/1(q_c) -> Display1/1, Body Rates Controller/2(q_ref)
  beta des (rad)/1 -> Ref Model and P Controller/1
  Longitudinal Controller: AoA or A_w_z/3(alpha_dot_c) -> Long Dyn Inversion: alpha_dot ->q/1(alpha_dot_c), Display/1
  AoA des (rad)/1 -> Longitudinal Controller: AoA or A_w_z/2(AoA des (rad))
  Anti-windup AoA/1 -> Longitudinal Controller: AoA or A_w_z/4(Anti-windup AoA)
  Anti-windup A_w_z/1 -> Longitudinal Controller: AoA or A_w_z/3(Anti-windup A_w_z)
  A_w_z des/1 -> Longitudinal Controller: AoA or A_w_z/1(A_w_z des)
  Sum/1 -> Display4/1, "Sigmoid "/1(In), Angular acc des/1  "v"
  Body Rates Controller/4(Angular acc des (rad/s^2)) -> Display3/1, Sum/2  "v_p+v_dot_ff"
  Bus Creator/1 -> On-line (adaptive) multi-layer NNs/3(NN variables)
  Memory/1 -> On-line (adaptive) multi-layer NNs/1(v_ad^ prev)
  Body Rates Controller/2(p_chanel vars) -> Bus Creator/2  "p_chanel_vars"
  Body Rates Controller/1(q_chanel vars) -> Bus Creator1/3  "q_chanel_vars"
  Longitudinal Controller: AoA or A_w_z/1(A_chanel vars) -> Bus Creator1/1  "A_chanel vars"
  Longitudinal Controller: AoA or A_w_z/2(alpha_chanel vars) -> Bus Creator1/2  "alpha_chanel vars"
  Bus Creator1/1 -> Bus Creator/1  "Long chanel"
  Ref Model and P Controller/2 -> Bus Creator2/1  "beta_sf_dot"
  Ref Model and P Controller/3 -> Sum1/1, Bus Creator2/2  "beta_sf"
  Sum1/1 -> Bus Creator2/3  "beta_err"
  Ref Model and P Controller/4 -> Sum1/2
  Ref Model and P Controller/5 -> Bus Creator2/4  "K_b_beta"
  Body Rates Controller/3(r_chanel vars) -> Bus Creator3/1  "r_chanel vars"
  Bus Creator2/1 -> Bus Creator3/2  "beta_chanel vars"
  Bus Creator3/1 -> Bus Creator/3  "beta_r_chanel"
  Anti-windup beta/1 -> Terminator1/1
  "Sigmoid "/1(Out) -> Memory/1
  On-line (adaptive) multi-layer NNs/1(v_ad^) -> Sum/1, Display2/1  "v_ad^"
  Ref Model and P Controller/1 -> Display5/1, Lat_dir Dyn Inversion: beta_dot->r_c/1(beta_dot_c)
  All measures/1 -> On-line (adaptive) multi-layer NNs/2(All_meas), Body Rates Controller/4(All_meas), Lat_dir Dyn Inversion: beta_dot->r_c/2(All_meas), Bus Selector3/1, Long Dyn Inversion: alpha_dot ->q/2(All_meas), Longitudinal Controller: AoA or A_w_z/5(All meas)
  Anti-windup signals/1 -> Terminator/1
  Ground/1 -> Control_in/1

== system F16ASYM_Controlled/Primary Controller/PI Primary Controller ==
  A_w_z des : Inport
  AoA des (rad) : Inport  Port=2
  p des (rad/s) : Inport  Port=3
  beta des (rad) : Inport  Port=4
  Anti-windup A_w_z : Inport  Port=5
  Anti-windup AoA : Inport  Port=6
  Anti-windup beta : Inport  Port=7
  All measures : Inport  Port=8
  Anti-windup signals : Inport  Port=9
  Body Rates Controller : Subsystem
  Bus Selector3 : BusSelector  OutputSignals=signal1.SS meas (rad)
  Display{,1..3} (4 alike) : Display
  Ground : Ground
  Lat_dir Dyn Inversion: beta_dot->r_c : Subsystem
  Long Dyn Inversion: alpha_dot ->q : Subsystem
  Longitudinal Controller: AoA or A_w_z : Subsystem  Variant=on  OverrideUsingVariant=Controller of A_w_z
  PI Controller: beta  controller : Adaptive_FaultTolerantControl/PI Controller  delta=0  K_a=0  y_i=trim_state(9)  Des_way=auto  omega_n=2  xi=1  Z1=-50  K_b=6  f_i=0.25  f_c=1
  Angular acc des : Outport
  Control_in : Outport  Port=2
  wires:
  A_w_z des/1 -> Longitudinal Controller: AoA or A_w_z/1(A_w_z des)
  Anti-windup A_w_z/1 -> Longitudinal Controller: AoA or A_w_z/3(Anti-windup A_w_z)
  Anti-windup AoA/1 -> Longitudinal Controller: AoA or A_w_z/4(Anti-windup AoA)
  AoA des (rad)/1 -> Longitudinal Controller: AoA or A_w_z/2(AoA des (rad))
  Longitudinal Controller: AoA or A_w_z/1(alpha_dot_c) -> Display/1, Long Dyn Inversion: alpha_dot ->q/1(alpha_dot_c)
  All measures/1 -> Bus Selector3/1, Lat_dir Dyn Inversion: beta_dot->r_c/2(All_meas), Body Rates Controller/4(All_meas), Longitudinal Controller: AoA or A_w_z/5(All meas), Long Dyn Inversion: alpha_dot ->q/2(All_meas)
  Anti-windup beta/1 -> PI Controller: beta  controller/3
  beta des (rad)/1 -> PI Controller: beta  controller/1
  Long Dyn Inversion: alpha_dot ->q/1(q_c) -> Body Rates Controller/2(q_ref), Display1/1
  p des (rad/s)/1 -> Body Rates Controller/1(p_ref)
  Body Rates Controller/1(Angular acc des (rad/s^2)) -> Angular acc des/1
  PI Controller: beta  controller/1 -> Lat_dir Dyn Inversion: beta_dot->r_c/1(beta_dot_c), Display3/1
  Anti-windup signals/1 -> Body Rates Controller/5(All Anti-windup signals)
  Bus Selector3/1 -> PI Controller: beta  controller/2  "<SS meas (rad)>"
  Lat_dir Dyn Inversion: beta_dot->r_c/1(r_c) -> Body Rates Controller/3(r_ref), Display2/1
  Ground/1 -> Control_in/1

== system F16ASYM_Controlled/SI and FDI/SI and FDI: Realistic ==
  note: RECONFIGURATION PARAMETERS
      |
      | 24. mass  Estimated mass
      | 25. S_current_L
      | 26. S_current_R
      | 27. S_fin_current
      | 28. x_cg
      | 29. Jy
      | 30. Jxz
      | 31. Jz
      | 32. Jx
      | 33. EFF_el_L
      | 34. EFF_el_R
      | 35. EFF_ail_L
      | 36. EFF_ail_R
      | 37. EFF_rud
      | 38. EFF_lef_L
      | 39. EFF_lef_R
      | 40. Delta_C_Lift_X
      | 41. Delta_C_Drag_X
      | 42. Delta_C_m_X
  Inexistent Reconfig bus : Inport
  Control comms : Inport  Port=2
  All  meas : Inport  Port=3
  Bus Creator : BusCreator  Inputs=3
  FDI: Assumed? : Subsystem  VariantControl=FDI: Realsitic
  Mass props : Selector  InputPortWidth=6  Indices=2:6
  Mux : Mux  Inputs=[9 7 3]
  Mux1 : Mux  Inputs=3
  SI : Subsystem
  mass : Selector  InputPortWidth=6
  Est reconf params : Outport
  wires:
  All  meas/1 -> SI/2(All meas), FDI: Assumed?/2(All  meas)
  FDI: Assumed?/3(Effectiveness) -> SI/1(Control Eff), Mux/2
  Mux/1 -> Bus Creator/3  "Reconfig signal"
  FDI: Assumed?/2(Blockades now) -> Bus Creator/2
  FDI: Assumed?/1(Blockades at) -> Bus Creator/1  "Blockades"
  Bus Creator/1 -> Est reconf params/1
  Inexistent Reconfig bus/1 -> FDI: Assumed?/1(Inexistent Reconfig bus)
  Control comms/1 -> FDI: Assumed?/3(Control comms), SI/3(Control comms)
  mass/1 -> Mux1/1
  SI/2(Est Surfs) -> Mux1/2
  Mass props/1 -> Mux1/3
  SI/1(Est Mass props) -> Mass props/1, mass/1
  Mux1/1 -> Mux/1
  SI/3(Est Aero changes) -> Mux/3

== system F16ASYM_Controlled/SI and FDI/SI and FDI: Unrealistic ==
  Inexistent Reconfig bus : Inport
  Control comms : Inport  Port=2
  All  meas : Inport  Port=3
  Terminator : Terminator
  Terminator1 : Terminator
  Est reconf params : Outport
  wires:
  Inexistent Reconfig bus/1 -> Est reconf params/1
  All  meas/1 -> Terminator/1
  Control comms/1 -> Terminator1/1
